simulink model "heat_balance_equation"  (R2023a)
settings: Solver=VariableStepAuto  StartTime=0.0  StopTime=10.0  RelTol=1e-3
model workspace (MAT data in the model file):
  J_p = 1
settings Model: Creator=2700783T  LastModifiedBy=2700783T

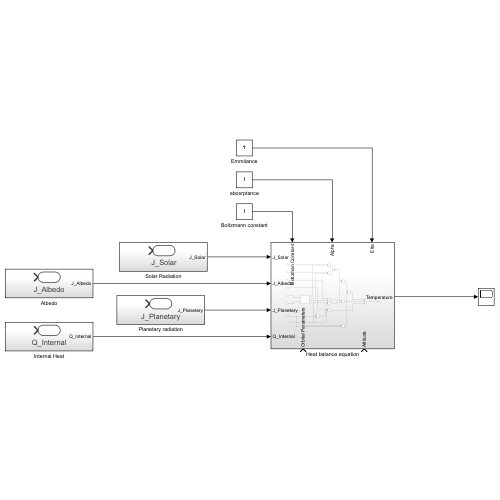
[thumbnail: Simulink's stored preview of the top-level diagram]
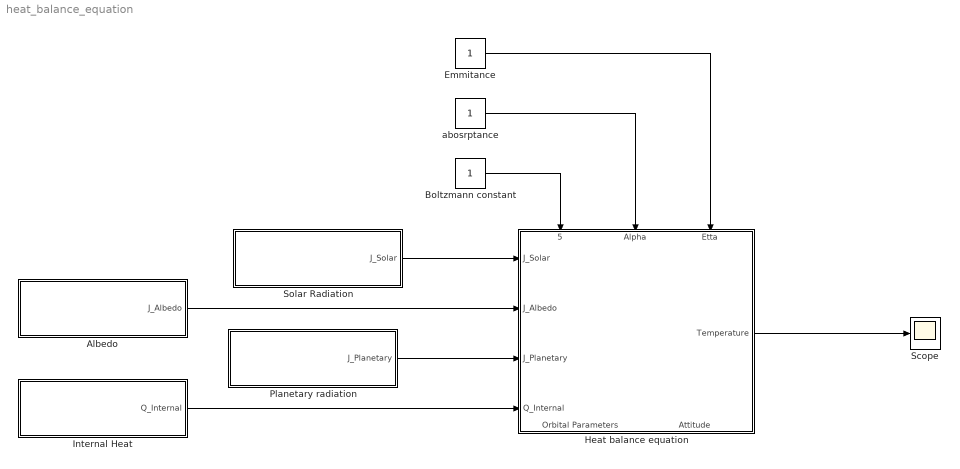
== system heat_balance_equation ==
  Albedo : Subsystem
  Boltzmann constant : Constant
  Emmitance : Constant
  Heat balance equation : Subsystem
      settings: PortSchema="{\"entries\":[{\"content\":{\"sides\":[{\"content\":{\"connectorIds\":[\"In1\",\"In2\",\"In3\",\"In4\"]},\"type\":\"ConnectorPlacement.EquallySpacedRectSide\",\"uuid\":\"a25b9e7a-7ff8-41a7-9f1d-c6a99f23b8fe\"},{\"content\":{\"connectorIds\":[\"Out1\"],\"side\":\"RIGHT\"},\"type\":\"ConnectorPlacement.EquallySpacedRectSide\",\"uuid\":\"d83a7c11-be56-4082-830d-8ef9d7a83d1c\"},{\"content\":{\"connectorIds\":[\"In5\",\"In6\",\"In7\"],\"side\":\"TOP\"},\"type\":\"ConnectorPlacement.EquallySpacedRectSide\",\"uuid\":\"eb98d061-36e6-4e05-921e-b89c3305e4a0\"},{\"content\":{\"connectorIds\":[\"In8\",\"In9\"],\"side\":\"BOTTOM\"},\"type\":\"ConnectorPlacement.EquallySpacedRectSide\",\"uuid\":\"53606723-e8b3-4c8b-930e-9844b9467044\"}]},\"type\":\"ConnectorPlacement.EquallySpacedConnector\",\"uuid\":\"34fae694-3bd9-43d0-ade2-1fca4a12a03c\"}],\"packageUris\":[\"http://schema.mathworks.com/mf0/Connector/R2020b\"],\"version\":\"1.0\"}"
  Internal Heat : Subsystem
  Planetary radiation : Subsystem
  Scope : Scope
  Solar Radiation : Subsystem
  abosrptance : Constant
  wires:
  Solar Radiation/1(J_Solar) -> Heat balance equation/1(J_Solar)
  Albedo/1(J_Albedo) -> Heat balance equation/2(J_Albedo)
  Planetary radiation/1(J_Planetary) -> Heat balance equation/3(J_Planetary)
  Internal Heat/1(Q_Internal) -> Heat balance equation/4(Q_Internal)
  Heat balance equation/1(Temperature) -> Scope/1
  Emmitance/1 -> Heat balance equation/7(Etta)
  abosrptance/1 -> Heat balance equation/6(Alpha)
  Boltzmann constant/1 -> Heat balance equation/5(Boltzman Constant)

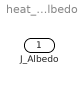
== system heat_balance_equation/Albedo ==
  J_Albedo : Outport

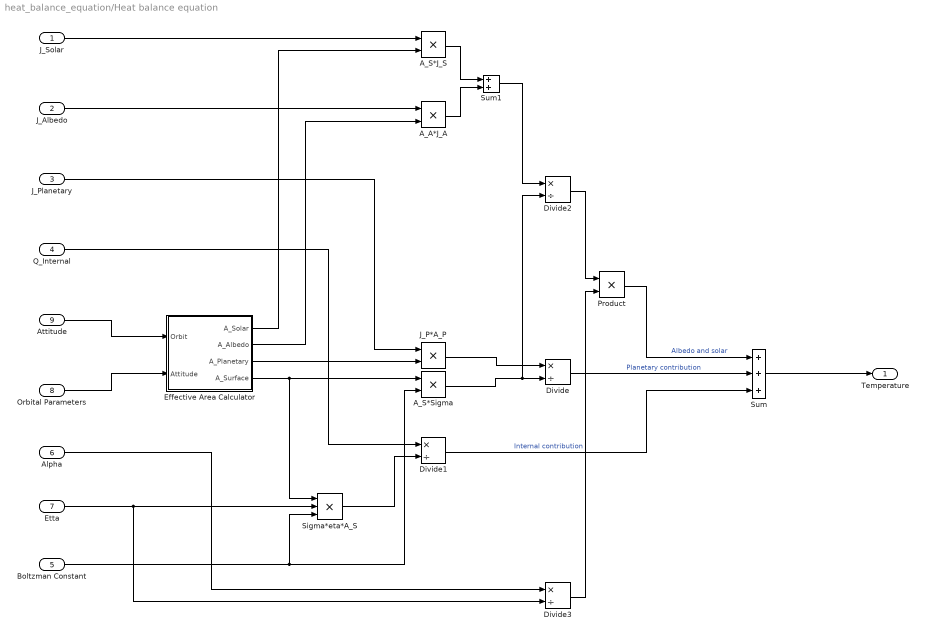
== system heat_balance_equation/Heat balance equation ==
  J_Solar : Inport
  J_Albedo : Inport  Port=2
  J_Planetary : Inport  Port=3
  Q_Internal : Inport  Port=4
  Boltzman Constant : Inport  Port=5
  Alpha : Inport  Port=6
  Etta : Inport  Port=7
  Orbital Parameters : Inport  Port=8
  Attitude : Inport  Port=9
  A_A*J_A : Product
  A_S*J_S : Product
  A_S*Sigma : Product
  Divide{,1..3} (4 alike) : Product  Inputs=*/
  Effective Area Calculator : Subsystem
  J_P*A_P : Product
  Product : Product
  Sigma*eta*A_S : Product  Inputs=3
  Sum : Sum  Inputs=+++
  Sum1 : Sum
  Temperature : Outport
  wires:
  Orbital Parameters/1 -> Effective Area Calculator/2(Attitude)
  Attitude/1 -> Effective Area Calculator/1(Orbit)
  J_P*A_P/1 -> Divide/1
  A_S*Sigma/1 -> Divide2/2, Divide/2
  Boltzman Constant/1 -> Sigma*eta*A_S/3, A_S*Sigma/2
  J_Planetary/1 -> J_P*A_P/1
  Effective Area Calculator/3(A_Planetary) -> J_P*A_P/2
  Effective Area Calculator/4(A_Surface) -> A_S*Sigma/1, Sigma*eta*A_S/1
  Divide/1 -> Sum/2  "Planetary contribution"
  Etta/1 -> Divide3/2, Sigma*eta*A_S/2
  Q_Internal/1 -> Divide1/1
  Sigma*eta*A_S/1 -> Divide1/2
  Divide1/1 -> Sum/3  "Internal contribution"
  J_Solar/1 -> A_S*J_S/1
  J_Albedo/1 -> A_A*J_A/1
  Effective Area Calculator/1(A_Solar) -> A_S*J_S/2
  Effective Area Calculator/2(A_Albedo) -> A_A*J_A/2
  A_S*J_S/1 -> Sum1/1
  A_A*J_A/1 -> Sum1/2
  Sum/1 -> Temperature/1
  Sum1/1 -> Divide2/1
  Alpha/1 -> Divide3/1
  Divide2/1 -> Product/1
  Divide3/1 -> Product/2
  Product/1 -> Sum/1  "Albedo and solar"

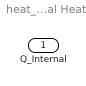
== system heat_balance_equation/Internal Heat ==
  Q_Internal : Outport

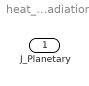
== system heat_balance_equation/Planetary radiation ==
  J_Planetary : Outport

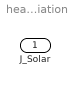
== system heat_balance_equation/Solar Radiation ==
  J_Solar : Outport

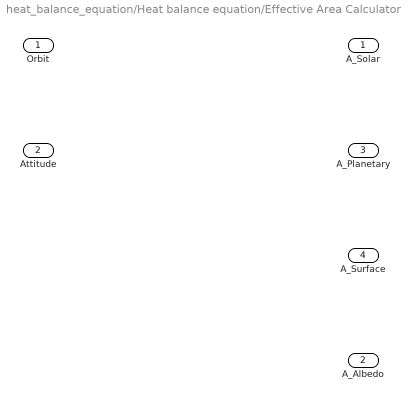
== system heat_balance_equation/Heat balance equation/Effective Area Calculator ==
  Orbit : Inport
  Attitude : Inport  Port=2
  A_Solar : Outport
  A_Albedo : Outport  Port=2
  A_Planetary : Outport  Port=3
  A_Surface : Outport  Port=4
